simulink subsystem "Compute_Lat_Err"  (R2022b)
settings: Solver=VariableStepAuto  StartTime=0.0  StopTime=10.0  RelTol=1e-3
settings Model: Creator=User  LastModifiedBy=User

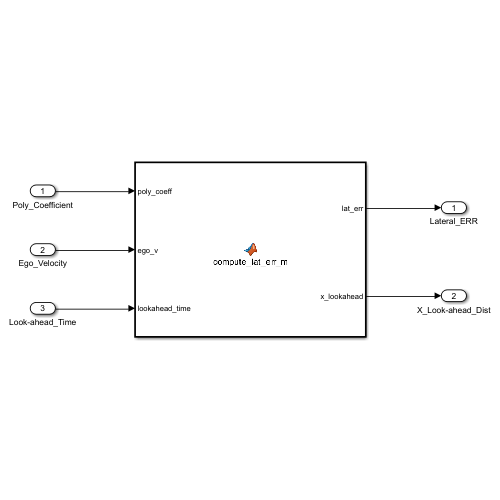
[thumbnail: Simulink's stored preview of the top-level diagram]
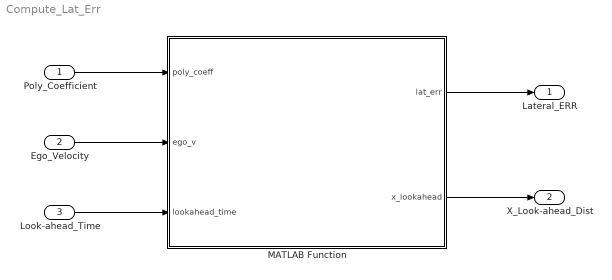
== system Compute_Lat_Err ==
  Poly_Coefficient : Inport
  Ego_Velocity : Inport  Port=2
  Look-ahead_Time : Inport  Port=3
  MATLAB Function : MATLAB Function  TreatAsAtomicUnit=on
  Lateral_ERR : Outport
  X_Look-ahead_Dist : Outport  Port=2
  wires:
  Poly_Coefficient/1 -> MATLAB Function/1(poly_coeff)
  Ego_Velocity/1 -> MATLAB Function/2(ego_v)
  Look-ahead_Time/1 -> MATLAB Function/3(lookahead_time)
  MATLAB Function/1(lat_err) -> Lateral_ERR/1
  MATLAB Function/2(x_lookahead) -> X_Look-ahead_Dist/1

== matlab function Compute_Lat_Err/MATLAB Function ==
  data: poly_coeff input; lat_err output; ego_v input; lookahead_time input; x_lookahead output
function [lat_err, x_lookahead] = compute_lat_err_m(poly_coeff, ego_v, lookahead_time)
    [lat_err, x_lookahead] = compute_lat_err(poly_coeff, ego_v, lookahead_time);
    
end
